simulink model "DCDCconverter"  (R2012b)
settings: Solver=ode3  StartTime=0.0  StopTime=inf  FixedStep=Tsample_simulink  RelTol=1e-3
PostLoadFcn:
  | , if any(exist('dsrtsu_mdlpostloadfcn', 'file') == [2, 3, 6]), try dsrtsu_mdlpostloadfcn('Execute', bdroot); catch fprintf('Error in PostLoadFcn (dsrtsu_mdlpostloadfcn) for model "%s":\n %s\n', bdroot, lasterr); end, end,
InitFcn:
  | load('../sim/me547_based_PI_controller_v3_saved_state.mat');
  | load('../sim/RuleBasedControlData_LiFe_76p8V_0C.mat');
undefined symbols (not defined in the file): BatVoltageLowerThresh, BatVoltageUpperThresh, C, DiscIntNeverNeededParam, Ea, fdesignblkfcn, gcbh, Icommand_Limit, Ireg_Integ_Limit, Kp_vc, MaxBatCurrent, MaxBatVoltage, MaxTemperature, MaxUCCurrent, MaxUCVoltage, Ra, RuleBasedControlHESSPowerValues, RuleBasedControlLUTValues, RuleBasedControlUCVoltageValues, TDelay_UltracapacitorRelay, Ts, Ts2, Tsample_simulink, UCVoltageLowerThresh, UCVoltageUpperThresh, Vbat, Vrail_rated
libraries: xpclib x35, rtilib1103 x8, dspsigops x5
(part 3 of 10)

== matlab function DCDCconverter/Test Icmd/Current_Profile_10Hz ==
  data: profile_on input; command_output output; simulation_time input
function command_output = generate_profile(profile_on, simulation_time)

persistent profile_on_condition index last_time period command profile;

if isempty(profile_on_condition)
    profile_on_condition = 5;
end
if isempty(index)
    index = 0;
end
if isempty(last_time)
    last_time = simulation_time;
end
if isempty(period)
    period = 1/10;
end
if isempty(command)
    command = 0;
end
if isempty(profile)
